simulink model "CreepMode_v2"  (R2022b)
settings: configuration reference "CommonModelConfiguration" (kept outside this file)
undefined symbols (not defined in the file): cc_param_13, cc_param_382
settings Model: Creator=vnarayan  LastModifiedBy=OTHOMSO1
settings ConfigSetRef: SourceName=CommonModelConfiguration  SourceLocation=Base Workspace

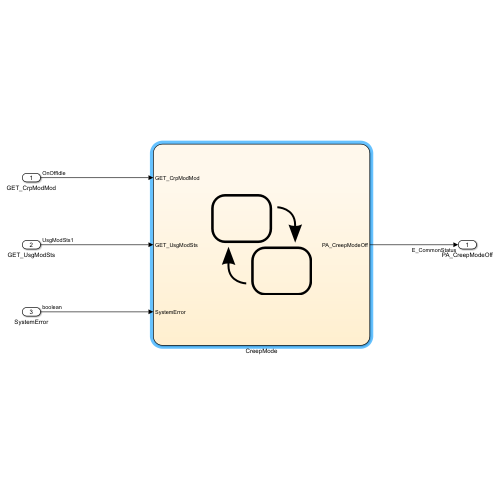
[thumbnail: Simulink's stored preview of the top-level diagram]
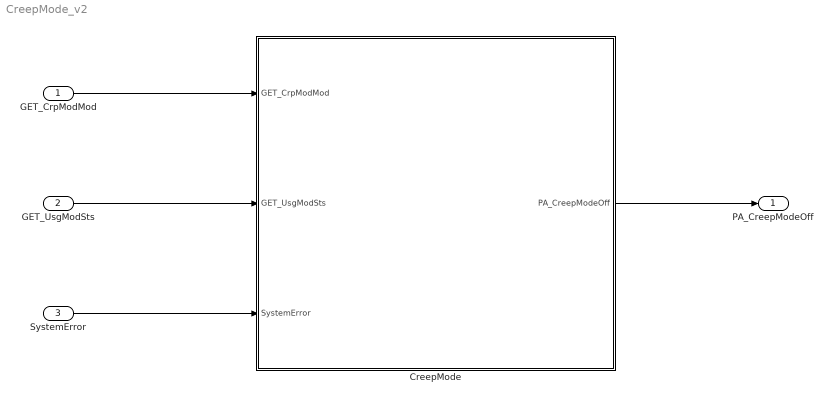
== system CreepMode_v2 ==
  GET_CrpModMod : Inport  OutDataTypeStr=Enum: OnOffIdle
  GET_UsgModSts : Inport  Port=2  OutDataTypeStr=Enum: UsgModSts1
  SystemError : Inport  Port=3  OutDataTypeStr=boolean
  CreepMode : Stateflow chart  TreatAsAtomicUnit=on
  PA_CreepModeOff : Outport  OutDataTypeStr=Enum: E_CommonStatus  BusOutputAsStruct=on
  wires:
  CreepMode/1(PA_CreepModeOff) -> PA_CreepModeOff/1
  GET_UsgModSts/1 -> CreepMode/2(GET_UsgModSts)
  SystemError/1 -> CreepMode/3(SystemError)
  GET_CrpModMod/1 -> CreepMode/1(GET_CrpModMod)

== stateflow chart CreepMode_v2/CreepMode ==
  state CARCONFIG_INVALID
    entry:
    PA_CreepModeOff = E_CommonStatus.NotPresent;
    note: 
  state SYSTEM_OK
    state activationCheck [function]
      (default) -> (junction 1067)
      (junction 1067) -> (junction 1070) [order 1] : [UsgModSts == UsgModSts1.UsgModSts1_UsgModDrvg ||...
          | UsgModSts == UsgModSts1.UsgModSts1_UsgModActv]
      (junction 1067) -> (junction 1075) [order 2] : {isActive = false;}
      (junction 1070) -> (junction 1071) : {isActive = true;}
      (junction 1071) -> (junction 1075)
    state NOT_ACTIVE
      entry:
      PA_CreepModeOff = E_CommonStatus.Disabled;
    state ACTIVE
      state OFF
        entry:
        PA_CreepModeOff = E_CommonStatus.Disabled;
      state ON
        entry:
        PA_CreepModeOff = E_CommonStatus.Available;
      (default) -> (junction 1142)
      (junction 1142) -> (junction 1143) [order 1] : [GET_CrpModMod==OnOffIdle.OnOffIdle_Off]
      (junction 1142) -> OFF [order 2]
      (junction 1143) -> ON
      OFF -> ON : [GET_CrpModMod==OnOffIdle.OnOffIdle_Off]
      ON -> OFF : [GET_CrpModMod==OnOffIdle.OnOffIdle_On]
    (default) -> (junction 131)
    (junction 131) -> NOT_ACTIVE [order 1] : [~activationCheck()]
    (junction 131) -> (junction 134) [order 2]
    NOT_ACTIVE -> ACTIVE : [activationCheck()]
    ACTIVE -> NOT_ACTIVE : [~activationCheck()]
    (junction 134) -> ACTIVE
  note: 
  note: 
  state SYSTEM_ERROR
    entry:
    PA_CreepModeOff = E_CommonStatus.SystemError;
  (default) -> (junction 1123)
  (junction 1123) -> CARCONFIG_INVALID [order 2]
  (junction 1123) -> (junction 137) [order 1] : [cc_param_382 == 4 &&...
      | cc_param_13 == 3]
  (junction 137) -> SYSTEM_OK [order 2]
  (junction 137) -> (junction 138) [order 1] : [SystemError == true]
  SYSTEM_ERROR -> SYSTEM_OK : [SystemError == false]
  SYSTEM_OK -> SYSTEM_ERROR : [SystemError == true]
  (junction 138) -> SYSTEM_ERROR
  data: PA_CreepModeOff output Enum: E_CommonStatus size=1; GET_CrpModMod input Enum: OnOffIdle; GET_UsgModSts input Enum: UsgModSts1; SystemError input boolean; cc_param_13 parameter; cc_param_382 parameter
